simulink model "V.1.0.SystemsmModelling"  (R2020a)
settings: Solver=ode23t  StartTime=0.0  StopTime=2000  MaxStep=2000.0  RelTol=1e-3
values from neighbouring files (symbols this model uses):
  InitialTemp = 300    [Setup.m]
undefined symbols (not defined in the file or in its folder): commanded_mass_flow, compressor_time_constant, condenser_length, copper_density, environment_temperature, evaporator_length, ground_temperature, max_throat_area, max_throat_temperature, min_throat_area, min_throat_temperature, pipe_diameter, pipe_thickness, target_temperature, temperature_delta, u_sat
libraries: fl_lib x208, refrigeration_lib x90, fl_ps_legacy_lib x50, nesl_utility x45
(part 3 of 7)

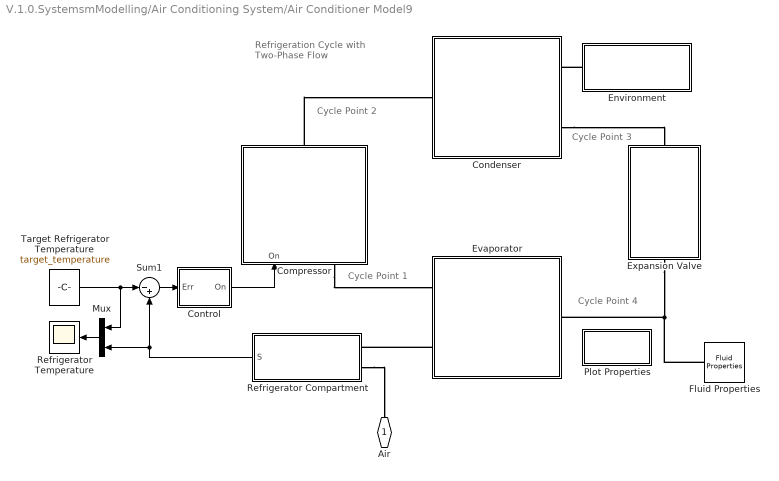
== system V.1.0.SystemsmModelling/Air Conditioning System/Air Conditioner Model9 ==
  note: Refrigeration Cycle
      | with Two-Phase Flow
  note: Cycle Point 1
  note: Cycle Point 3
  note: Cycle Point 2
  note: Cycle Point 4
  Compressor : Subsystem
      mask Display:
      | % Fading color
      | % Center to right
      | patch(sin(0.00*pi:0.05:1.10*pi),cos(0.00*pi:0.05:1.10*pi),[1;0.90;0.94]);
      | patch(sin(0.05*pi:0.05:0.95*pi),cos(0.05*pi:0.05:0.95*pi),[1;0.85;0.88]);
      | patch(sin(0.10*pi:0.05:0.90*pi),cos(0.10*pi:0.05:0.90*pi),[1;0.80;0.82]);
      | patch(sin(0.15*pi:0.05:0.85*pi),cos(0.15*pi:0.05:0.85*pi),[1;0.75;0.76]);
      | patch(sin(0.20*pi:0.05:0.80*pi),cos(0.20*pi:0.05:0.80*pi),[1;0.70;0.70]);
      | % Center to left
      | patch(sin(1.00*pi:0.05:2.00*pi),cos(1.00*pi:0.05:2.00*pi),[0.94;0.90;1]);
      | patch(sin(1.05*pi:0.05:1.95*pi),cos(1.05*pi:0.05:1.95*pi),[0.88;0.90;1]);
      | patch(sin(1.10*pi:0.05:1.90*pi),cos(1.10*pi:0.05:1.90*pi),[0.82;0.90;1]);
      | patch(sin(1.15*pi:0.05:1.85*pi),cos(1.15*pi:0.05:1.85*pi),[0.76;0.90;1]);
      | patch(sin(1.20*pi:0.05:1.80*pi),cos(1.20*pi:0.05:1.80*pi),[0.70;0.90;1]);
      | % Circle
      | plot(sin(0:0.1:2.2*pi),cos(0:0.1:2.2*pi));
      | % Angled lines
      | plot(sin([-0.6*pi/3 3.6*pi/8]),cos([-0.6*pi/3 3.6*pi/8]));
      | plot(sin([-0.6*pi/3 3.6*pi/8]),-cos([-0.6*pi/3 3.6*pi/8]));
      | plot(1.15*sin([-pi/4 3*pi/4]),1.15*cos([-pi/4 3*pi/4]));
      | % Arrow
      | patch([1.15*sin(-pi/4)+0.01;1.15*sin(3*pi/4)+0.01;1.15*sin(3*pi/4)-0.01;1.15*sin(-pi/4)-0.01],[1.15*cos(-pi/4)+0.01;1.15*cos(3*pi/4)+0.01;1.15*cos(3*pi/4)-0.01;1.15*cos(-pi/4)-0.01],[0;0;0])
      | patch([0.8*sin(3*pi/4)+0.05;1.15*sin(3*pi/4)+0.00;1.15*sin(3*pi/4)-0.00;0.8*sin(3*pi/4)-0.05],[0.8*cos(3*pi/4)+0.05;1.15*cos(3*pi/4)+0.00;1.15*cos(3*pi/4)-0.00;0.8*cos(3*pi/4)-0.05],[0;0;0])
      | % Points to set range for plotting area
      | color('white');plot(1.3,1.3);plot(-1.3,-1.3)
      | color('black');
      | 
      | port_label('LConn',1,'A');
      | port_label('RConn',1,'B');
      | port_label('input',1,'On');
  Condenser : Subsystem
      mask Display:
      | % Colored patches
      | % Center to right
      | patch(sin(0.0*pi:0.05:1.1*pi),cos(0.0*pi:0.05:1.1*pi),[1;0.58;0.58]);
      | patch(sin(0.1*pi:0.05:0.9*pi),cos(0.1*pi:0.05:0.9*pi),[1;0.64;0.64]);
      | patch(sin(0.2*pi:0.05:0.8*pi),cos(0.2*pi:0.05:0.8*pi),[1;0.70;0.70]);
      | % Center to left
      | patch(sin(1.0*pi:0.05:2.0*pi),cos(1.0*pi:0.05:2.0*pi),[1;0.52;0.52]);
      | patch(sin(1.1*pi:0.05:1.9*pi),cos(1.1*pi:0.05:1.9*pi),[1;0.46;0.46]);
      | patch(sin(1.2*pi:0.05:1.8*pi),cos(1.2*pi:0.05:1.8*pi),[1;0.40;0.40]);
      | % Circle
      | plot(sin(0:0.1:2.2*pi),cos(0:0.1:2.2*pi));
      | % 'M'
      | plot([0.5 0.5],[-1.2 0.5]);
      | plot([-0.5 -0.5],[-1.2 0.5]);
      | plot([0.5 0],[0.5 -0.2]);
      | plot([-0.5 0],[0.5 -0.2]);
      | % Plot points to set plot range
      | color('white');plot(1.3,1.3);plot(-1.3,-1.3)
      | color('black');
      | 
      | port_label('RConn',1,'A');
      | port_label('LConn',1,'T');
      | port_label('LConn',2,'B');
  Control : Subsystem
  Environment : Subsystem
      mask Display:
      | % Colored patch
      | patch([sin(0:0.1:1*pi)*0.25+0.4 sin(pi:0.1:2*pi)*0.25-0.4],[cos(0:0.1:1*pi) cos(pi:0.1:2*pi)],[1;0.9;0.9]);
      | % Outer rounded rectangle
      | plot(sin(0:0.1:1*pi)*0.25+0.4,cos(0:0.1:1*pi));
      | plot(sin(pi:0.1:2*pi)*0.25-0.4,cos(pi:0.1:2*pi));
      | plot([-0.4 0.4],[1 1]);
      | plot([-0.4 0.4],[-1 -1]);
      | % House frame
      | plot([-0.3 -0.3],[-0.866,0.866*0.2])
      | plot([0.3 0.3],[-0.866,0.866*0.2])
      | plot([0.3 0],[0.866*0.2, 0.866])
      | plot([-0.3 0],[0.866*0.2, 0.866])
      | plot([-0.3 0.3],[-0.866 -0.866])
      | plot([-0.3 0.3],[0.866 0.866]*0.2)
      | plot([-0.2 -0.04],[0.866 0.866]*0)
      | % Window
      | plot([-0.2 -0.04],[-1 -1]*0.2)
      | plot([-0.2 -0.04],[-1 -1]*0.4)
      | plot([-0.2 -0.2],[0 -0.4])
      | plot([-0.12 -0.12],[0 -0.4])
      | plot([-0.04 -0.04],[0 -0.4])
      | % Door
      | plot([0.05 0.05],[-0.866 -0.2])
      | plot([0.18 0.18],[-0.866 -0.2])
      | plot([0.05 0.18],[-0.2 -0.2])
      | patch([0.12 0.15 0.12 0.15],[-0.5 -0.5 -0.54 -0.54],[0;0;0])
      | % Outer boundary (so plot labels are visible)
      | color('white');plot(0.8660,0.8660);plot(-0.8660,-0.8660)
      | color('black');
      | port_label('LConn',1,'T');
  Evaporator : Subsystem
      mask Display:
      | % Fading color
      | % Center to right
      | patch(sin(0.00*pi:0.05:1.10*pi),cos(0.00*pi:0.05:1.10*pi),[0.58;0.70;1]);
      | patch(sin(0.05*pi:0.05:0.95*pi),cos(0.05*pi:0.05:0.95*pi),[0.63;0.75;1]);
      | patch(sin(0.10*pi:0.05:0.90*pi),cos(0.10*pi:0.05:0.90*pi),[0.66;0.80;1]);
      | patch(sin(0.15*pi:0.05:0.85*pi),cos(0.15*pi:0.05:0.85*pi),[0.69;0.85;1]);
      | patch(sin(0.20*pi:0.05:0.80*pi),cos(0.20*pi:0.05:0.80*pi),[0.70;0.90;1]);
      | % Center to left
      | patch(sin(1.00*pi:0.05:2.00*pi),cos(1.00*pi:0.05:2.00*pi),[0.52;0.60;1]);
      | patch(sin(1.05*pi:0.05:1.95*pi),cos(1.05*pi:0.05:1.95*pi),[0.49;0.55;1]);
      | patch(sin(1.10*pi:0.05:1.90*pi),cos(1.10*pi:0.05:1.90*pi),[0.46;0.50;1]);
      | patch(sin(1.15*pi:0.05:1.85*pi),cos(1.15*pi:0.05:1.85*pi),[0.43;0.45;1]);
      | patch(sin(1.20*pi:0.05:1.80*pi),cos(1.20*pi:0.05:1.80*pi),[0.40;0.40;1]);
      | % Circle
      | plot(sin(0:0.1:2.2*pi),cos(0:0.1:2.2*pi));
      | % 'M'
      | plot([0.5 0.5],[-1.2 0.5]);
      | plot([-0.5 -0.5],[-1.2 0.5]);
      | plot([0.5 0],[0.5 -0.2]);
      | plot([-0.5 0],[0.5 -0.2]);
      | % Plot points to set plotting range
      | color('white');plot(1.3,1.3);plot(-1.3,-1.3)
      | color('black');
      | 
      | port_label('LConn',1,'A');
      | port_label('RConn',1,'B');
      | port_label('RConn',2,'T');
  Expansion Valve : Subsystem
      mask Display:
      | % Colored patches
      | patch([-1 -1 0],[0.5 -0.5 0],[1;0.4;0.4]);
      | patch([1 1 0],[0.5 -0.5 0],[0.4;0.4;1]);
      | % Valve
      | plot([1 1],[0.5 -0.5]);
      | plot([-1 -1],[0.5 -0.5]);
      | plot([-1 1],[0.5 -0.5]);
      | plot([-1 1],[-0.5 0.5]);
      | % Arrow
      | patch([1.15*sin(-pi/4-0.01);1.15*sin(-pi/4+0.01);1*sin(3*pi/4-0.01);1*sin(3*pi/4+0.01)],[1.15*cos(-pi/4-0.01);1.15*cos(-pi/4+0.01);1*cos(3*pi/4-0.01);1*cos(3*pi/4+0.01)],[0;0;0])
      | patch([0.8*sin(3*pi/4+0.07);1.15*sin(3*pi/4+0.00);1.15*sin(3*pi/4-0.00);0.8*sin(3*pi/4-0.07)],[0.8*cos(3*pi/4+0.07);1.15*cos(3*pi/4+0.00);1.15*cos(3*pi/4-0.00);0.8*cos(3*pi/4-0.07)],[0;0;0])
      | % Plot outer points to set plot range
      | color('white'); plot(-1.3,0); plot(1.3,0);
      | color('black');
      | port_label('LConn',1,'A');
      | port_label('RConn',1,'B');
  Fluid Properties : refrigeration_lib/Fluid Properties  p_TLU=p_TLU MPa  u_TLU=u_TLU kJ/kg  v_TLU=v_TLU m^3/kg  T_TLU=T_TLU K  mu_TLU=mu_TLU s*uPa  k_TLU=k_TLU W/(m*K)  Pr_TLU=Pr_TLU  u_liq=u_sat(:,1) kJ/kg  u_vap=u_sat(:,2) kJ/kg
      settings: InternalSimscapePortConfiguration="{\"Bottom\":[],\"Left\":[],\"Right\":[{\"id\":\"A\",\"label\":\"\",\"type\":\"refrigeration.refrigeration\"}],\"Top\":[]}"
  Mux : Mux  Inputs=2
  Plot Properties : Subsystem
      settings: OpenFcn=plotFluidProperties()
      mask Display: disp('Plot Fluid\nProperties');
  Refrigerator Compartment : Subsystem
      mask Display:
      | % Color
      | patch([sin(0:0.1:1*pi)*0.25+0.4 sin(pi:0.1:2*pi)*0.25-0.4],[cos(0:0.1:1*pi) cos(pi:0.1:2*pi)],[0.70;0.90;1]);
      | % Outer rounded rectangle
      | plot(sin(pi:0.1:2*pi)*0.25-0.4,cos(pi:0.1:2*pi));
      | plot(sin(0:0.1:1*pi)*0.25+0.4,cos(0:0.1:1*pi));
      | plot(sin(pi:0.1:2*pi)*0.25-0.4,cos(pi:0.1:2*pi));
      | plot([-0.4 0.4],[1 1]);
      | plot([-0.4 0.4],[-1 -1]);
      | % Outer points to set size of plot range
      | color('white');plot(0.8660,0.8660);plot(-0.8660,-0.8660)
      | color('black');
      | % Snowflake
      | plot([0 0],[0.8 -0.8]);
      | plot([0 0.1],[0.5 0.7]);
      | plot([0 -0.1],[0.5 0.7]);
      | plot([0 0.1],[-0.5 -0.7]);
      | plot([0 -0.1],[-0.5 -0.7]);
      | plot(0.3*sin([pi/3 4*pi/3]),1*cos([pi/3 4*pi/3]));
      | plot([0.22*sin(pi/3) 0.25*sin(pi/4)],[0.7*cos(pi/3) 0.84*cos(pi/4)]);
      | plot([0.22*sin(pi/3) 0.25*sin(pi/2)],[0.7*cos(pi/3) 0.325*cos(pi/4)]);
      | plot([0.22*sin(pi/3) 0.25*sin(pi/4)],[-0.7*cos(pi/3) -0.84*cos(pi/4)]);
      | plot([0.22*sin(pi/3) 0.25*sin(pi/2)],[-0.7*cos(pi/3) -0.325*cos(pi/4)]);
      | plot(-0.3*sin([pi/3 4*pi/3]),1*cos([pi/3 4*pi/3]));
      | plot([-0.22*sin(pi/3) -0.25*sin(pi/4)],[0.7*cos(pi/3) 0.84*cos(pi/4)]);
      | plot([-0.22*sin(pi/3) -0.25*sin(pi/2)],[0.7*cos(pi/3) 0.325*cos(pi/4)]);
      | plot([-0.22*sin(pi/3) -0.25*sin(pi/4)],[-0.7*cos(pi/3) -0.84*cos(pi/4)]);
      | plot([-0.22*sin(pi/3) -0.25*sin(pi/2)],[-0.7*cos(pi/3) -0.325*cos(pi/4)]);
      | plot([0 0.1],[-0.5 -0.7]);
      | plot([0 -0.1],[-0.5 -0.7]);
      | % Labels
      | port_label('LConn',1,'T');
      | port_label('output',1,'S');
  Refrigerator Temperature : Scope
  Sum1 : Sum  Inputs=|-+
  Target Refrigerator Temperature : Constant  Value=target_temperature
  Air : PMIOPort  Side=Left
  wires:
  Control/1(On) -> Compressor/1(On)
  Refrigerator Compartment/1(S) -> Mux/2, Sum1/2
  Target Refrigerator Temperature/1 -> Sum1/1, Mux/1
  Mux/1 -> Refrigerator Temperature/1
  Sum1/1 -> Control/1(Err)
  connections:
  Expansion Valve/RConn1 -- Fluid Properties/RConn1 -- Evaporator/LConn1
  Environment/LConn1 -- Condenser/LConn1
  Evaporator/RConn2 -- Refrigerator Compartment/LConn1
  Compressor/LConn1 -- Evaporator/RConn1
  Condenser/LConn2 -- Expansion Valve/LConn1
  Compressor/RConn1 -- Condenser/RConn1
  Refrigerator Compartment/LConn2 -- Air/RConn1

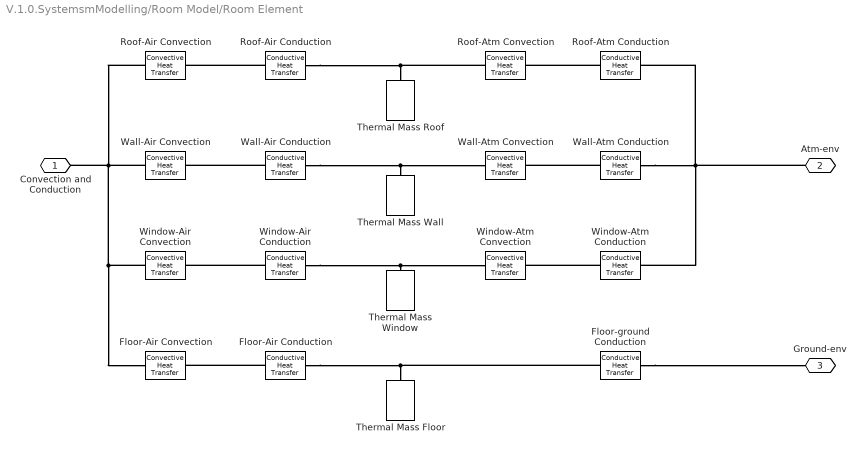
== system V.1.0.SystemsmModelling/Room Model/Room Element  ==
  " Wall-Air Conduction" : fl_lib/Thermal/Thermal Elements/Conductive Heat Transfer  area=375 m^2  thickness=0.2 m  th_cond=0.15 W/(m*K)  T_specify=off  T_priority=None  T=0 K  T_nominal_specify=off  T_nominal_unit=K  T_nominal_value=1  Q_specify=off  Q_priority=None  Q=0 W  Q_nominal_specify=off  Q_nominal_unit=W  Q_nominal_value=1
  " Wall-Atm Conduction" : fl_lib/Thermal/Thermal Elements/Conductive Heat Transfer  area=375 m^2  thickness=0.2 m  th_cond=0.15 W/(m*K)  T_specify=off  T_priority=None  T=0 K  T_nominal_specify=off  T_nominal_unit=K  T_nominal_value=1  Q_specify=off  Q_priority=None  Q=0 W  Q_nominal_specify=off  Q_nominal_unit=W  Q_nominal_value=1
  " Window-Air Conduction" : fl_lib/Thermal/Thermal Elements/Conductive Heat Transfer  area=25 m^2  thickness=0.2 m  th_cond=0.96 W/(m*K)  T_specify=off  T_priority=None  T=0 K  T_nominal_specify=off  T_nominal_unit=K  T_nominal_value=1  Q_specify=off  Q_priority=None  Q=0 W  Q_nominal_specify=off  Q_nominal_unit=W  Q_nominal_value=1
  " Window-Atm Conduction" : fl_lib/Thermal/Thermal Elements/Conductive Heat Transfer  area=25 m^2  thickness=0.2 m  th_cond=0.96 W/(m*K)  T_specify=off  T_priority=None  T=0 K  T_nominal_specify=off  T_nominal_unit=K  T_nominal_value=1  Q_specify=off  Q_priority=None  Q=0 W  Q_nominal_specify=off  Q_nominal_unit=W  Q_nominal_value=1
  Floor-Air Conduction : fl_lib/Thermal/Thermal Elements/Conductive Heat Transfer  area=25 m^2  thickness=0.2 m  th_cond=0.96 W/(m*K)  T_specify=off  T_priority=None  T=0 K  T_nominal_specify=off  T_nominal_unit=K  T_nominal_value=1  Q_specify=off  Q_priority=None  Q=0 W  Q_nominal_specify=off  Q_nominal_unit=W  Q_nominal_value=1
  Floor-Air Convection : fl_lib/Thermal/Thermal Elements/Convective Heat Transfer  area=20 m^2  heat_tr_coeff=3.3 W/(m^2 * K)  T_specify=off  T_priority=None  T=0 K  T_nominal_specify=off  T_nominal_unit=K  T_nominal_value=1  Q_specify=off  Q_priority=None  Q=0 W  Q_nominal_specify=off  Q_nominal_unit=W  Q_nominal_value=1
  Floor-ground Conduction : fl_lib/Thermal/Thermal Elements/Conductive Heat Transfer  area=25 m^2  thickness=0.2 m  th_cond=0.96 W/(m*K)  T_specify=off  T_priority=None  T=0 K  T_nominal_specify=off  T_nominal_unit=K  T_nominal_value=1  Q_specify=off  Q_priority=None  Q=0 W  Q_nominal_specify=off  Q_nominal_unit=W  Q_nominal_value=1
  Roof-Air Conduction : fl_lib/Thermal/Thermal Elements/Conductive Heat Transfer  area=100 m^2  thickness=0.2 m  th_cond=0.12 W/(m*K)  T_specify=off  T_priority=None  T=0 K  T_nominal_specify=off  T_nominal_unit=K  T_nominal_value=1  Q_specify=off  Q_priority=None  Q=0 W  Q_nominal_specify=off  Q_nominal_unit=W  Q_nominal_value=1
  Roof-Air Convection : fl_lib/Thermal/Thermal Elements/Convective Heat Transfer  area=100 m^2  heat_tr_coeff=20 W/(m^2 * K)  T_specify=off  T_priority=None  T=0 K  T_nominal_specify=off  T_nominal_unit=K  T_nominal_value=1  Q_specify=off  Q_priority=None  Q=0 W  Q_nominal_specify=off  Q_nominal_unit=W  Q_nominal_value=1
  Roof-Atm Conduction : fl_lib/Thermal/Thermal Elements/Conductive Heat Transfer  area=100 m^2  thickness=0.2 m  th_cond=0.12 W/(m*K)  T_specify=off  T_priority=None  T=0 K  T_nominal_specify=off  T_nominal_unit=K  T_nominal_value=1  Q_specify=off  Q_priority=None  Q=0 W  Q_nominal_specify=off  Q_nominal_unit=W  Q_nominal_value=1
  Roof-Atm Convection : fl_lib/Thermal/Thermal Elements/Convective Heat Transfer  area=100 m^2  heat_tr_coeff=20 W/(m^2 * K)  T_specify=off  T_priority=None  T=0 K  T_nominal_specify=off  T_nominal_unit=K  T_nominal_value=1  Q_specify=off  Q_priority=None  Q=0 W  Q_nominal_specify=off  Q_nominal_unit=W  Q_nominal_value=1
  Thermal Mass Floor : fl_lib/Thermal/Thermal Elements/Thermal Mass  mass=48 kg  sp_heat=840.7 J/kg/K  T_specify=on  T_priority=High  T=InitialTemp K  T_nominal_specify=off  T_nominal_unit=K  T_nominal_value=1  Q_specify=off  Q_priority=None  Q=0 W  Q_nominal_specify=off  Q_nominal_unit=W  Q_nominal_value=1
  Thermal Mass Roof : fl_lib/Thermal/Thermal Elements/Thermal Mass  mass=48 kg  sp_heat=853.7 J/kg/K  T_specify=on  T_priority=High  T=InitialTemp K  T_nominal_specify=off  T_nominal_unit=K  T_nominal_value=1  Q_specify=off  Q_priority=None  Q=0 W  Q_nominal_specify=off  Q_nominal_unit=W  Q_nominal_value=1
  Thermal Mass Wall : fl_lib/Thermal/Thermal Elements/Thermal Mass  mass=180 kg  sp_heat=868.2 J/kg/K  T_specify=on  T_priority=High  T=InitialTemp K  T_nominal_specify=off  T_nominal_unit=K  T_nominal_value=1  Q_specify=off  Q_priority=None  Q=0 W  Q_nominal_specify=off  Q_nominal_unit=W  Q_nominal_value=1
  Thermal Mass Window : fl_lib/Thermal/Thermal Elements/Thermal Mass  mass=11 kg  sp_heat=840 J/kg/K  T_specify=on  T_priority=High  T=InitialTemp K  T_nominal_specify=off  T_nominal_unit=K  T_nominal_value=1  Q_specify=off  Q_priority=None  Q=0 W  Q_nominal_specify=off  Q_nominal_unit=W  Q_nominal_value=1
  Wall-Air Convection : fl_lib/Thermal/Thermal Elements/Convective Heat Transfer  area=375 m^2  heat_tr_coeff=20 W/(m^2 * K)  T_specify=off  T_priority=None  T=0 K  T_nominal_specify=off  T_nominal_unit=K  T_nominal_value=1  Q_specify=off  Q_priority=None  Q=0 W  Q_nominal_specify=off  Q_nominal_unit=W  Q_nominal_value=1
  Wall-Atm Convection : fl_lib/Thermal/Thermal Elements/Convective Heat Transfer  area=375 m^2  heat_tr_coeff=20 W/(m^2 * K)  T_specify=off  T_priority=None  T=0 K  T_nominal_specify=off  T_nominal_unit=K  T_nominal_value=1  Q_specify=off  Q_priority=None  Q=0 W  Q_nominal_specify=off  Q_nominal_unit=W  Q_nominal_value=1
  Window-Air Convection : fl_lib/Thermal/Thermal Elements/Convective Heat Transfer  area=25 m^2  heat_tr_coeff=3.3 W/(m^2 * K)  T_specify=off  T_priority=None  T=0 K  T_nominal_specify=off  T_nominal_unit=K  T_nominal_value=1  Q_specify=off  Q_priority=None  Q=0 W  Q_nominal_specify=off  Q_nominal_unit=W  Q_nominal_value=1
  Window-Atm Convection : fl_lib/Thermal/Thermal Elements/Convective Heat Transfer  area=25 m^2  heat_tr_coeff=3.3 W/(m^2 * K)  T_specify=off  T_priority=None  T=0 K  T_nominal_specify=off  T_nominal_unit=K  T_nominal_value=1  Q_specify=off  Q_priority=None  Q=0 W  Q_nominal_specify=off  Q_nominal_unit=W  Q_nominal_value=1
  Convection and Conduction : PMIOPort  Side=Left
  Atm-env : PMIOPort  Port=2  Side=Left
  Ground-env : PMIOPort  Port=3  Side=Left
  connections:
  " Window-Atm Conduction"/RConn1 -- Window-Atm Convection/LConn1
  Floor-ground Conduction/LConn1 -- Ground-env/RConn1
  Roof-Air Conduction/RConn1 -- Roof-Air Convection/LConn1
  Floor-Air Conduction/LConn1 -- Floor-ground Conduction/RConn1 -- Thermal Mass Floor/LConn1
  " Wall-Atm Conduction"/LConn1 -- Atm-env/RConn1 -- Roof-Atm Conduction/LConn1 -- " Window-Atm Conduction"/LConn1
  Roof-Air Convection/RConn1 -- Convection and Conduction/RConn1 -- Window-Air Convection/RConn1 -- Floor-Air Convection/RConn1 -- Wall-Air Convection/RConn1
  Roof-Atm Convection/RConn1 -- Roof-Air Conduction/LConn1 -- Thermal Mass Roof/LConn1
  Roof-Atm Conduction/RConn1 -- Roof-Atm Convection/LConn1
  " Wall-Air Conduction"/LConn1 -- Wall-Atm Convection/RConn1 -- Thermal Mass Wall/LConn1
  " Window-Air Conduction"/LConn1 -- Window-Atm Convection/RConn1 -- Thermal Mass Window/LConn1
  " Wall-Atm Conduction"/RConn1 -- Wall-Atm Convection/LConn1
  " Wall-Air Conduction"/RConn1 -- Wall-Air Convection/LConn1
  " Window-Air Conduction"/RConn1 -- Window-Air Convection/LConn1
  Floor-Air Conduction/RConn1 -- Floor-Air Convection/LConn1

== system V.1.0.SystemsmModelling/Air Conditioning System/Air Conditioner Model/Compressor ==
  On : Inport
  Commanded Mass Flow Rate : Gain  Gain=commanded_mass_flow
  Compressor Lag : TransferFcn  Numerator=[(9/compressor_time_constant)^2]  Denominator=[1, 2*(9/compressor_time_constant), (9/compressor_time_constant)^2]
  Controlled Mass Flow Rate Source : refrigeration_lib/Controlled Mass Flow Rate Source  S=pi*pipe_diameter^2/4 m^2  L=0.1 m  mdot_specify=off  mdot_priority=High  mdot=0 kg/s  mdot_nominal_specify=off  mdot_nominal_unit=kg/s  mdot_nominal_value=1  phi_A_specify=off  phi_A_priority=High  phi_A=0 kW  phi_A_nominal_specify=off  phi_A_nominal_unit=kW  phi_A_nominal_value=1  phi_B_specify=off  phi_B_priority=High  phi_B=0 kW  phi_B_nominal_specify=off  phi_B_nominal_unit=kW  phi_B_nominal_value=1  u_AI_specify=off  u_AI_priority=High  u_AI=396.921741345 kJ/kg  u_AI_nominal_specify=off  u_AI_nominal_unit=kJ/kg  u_AI_nominal_value=1  v_A_specify=off  v_A_priority=High  v_A=0.230606289431 m^3/kg  v_A_nominal_specify=off  v_A_nominal_unit=m^3/kg  v_A_nominal_value=1  u_BI_specify=off  u_BI_priority=High  u_BI=396.921741345 kJ/kg  u_BI_nominal_specify=off  u_BI_nominal_unit=kJ/kg  u_BI_nominal_value=1  v_B_specify=off  v_B_priority=High  v_B=0.230606289431 m^3/kg  v_B_nominal_specify=off  v_B_nominal_unit=m^3/kg  v_B_nominal_value=1  u_2_specify=off  u_2_priority=High  u_2=396.921741345 kJ/kg  u_2_nominal_specify=off  u_2_nominal_unit=kJ/kg  u_2_nominal_value=1  u_3_specify=off  u_3_priority=High  u_3=396.921741345 kJ/kg  u_3_nominal_specify=off  u_3_nominal_unit=kJ/kg  u_3_nominal_value=1
      settings: InternalSimscapePortConfiguration="{\"Bottom\":[],\"Left\":[{\"id\":\"A\",\"label\":\"A\",\"type\":\"refrigeration.refrigeration\"},{\"id\":\"M\",\"label\":\"M\",\"type\":\"input\"}],\"Right\":[{\"id\":\"B\",\"label\":\"B\",\"type\":\"refrigeration.refrigeration\"},{\"id\":\"W\",\"label\":\"W\",\"type\":\"output\"}],\"Top\":[]}"
  Simulink-PS Converter : nesl_utility/Simulink-PS Converter  PhysicalDomain=network_engine_domain  SubClassName=ps_input  LeftPortType=input  RightPortType=output  PseudoPeriodic=off  Frequencies=[]  NoiseDistribution=none  NoiseParameters=[]  Unit=kg/s  AffineConversion=off  FilteringAndDerivatives=zero  SimscapeFilterOrder=1  InputFilterTimeConstant=0.001  UdotUserProvided=1
  B : PMIOPort  Side=Right
  A : PMIOPort  Port=2  Side=Left
  wires:
  Compressor Lag/1 -> Simulink-PS Converter/1
  Commanded Mass Flow Rate/1 -> Compressor Lag/1
  On/1 -> Commanded Mass Flow Rate/1
  connections:
  Controlled Mass Flow Rate Source/RConn1 -- B/RConn1
  Controlled Mass Flow Rate Source/LConn2 -- Simulink-PS Converter/RConn1
  A/RConn1 -- Controlled Mass Flow Rate Source/LConn1

== system V.1.0.SystemsmModelling/Air Conditioning System/Air Conditioner Model/Condenser ==
  Condenser Conduction : fl_lib/Thermal/Thermal Elements/Conductive Heat Transfer  area=pi*pipe_diameter*condenser_length m^2  thickness=pipe_thickness m  th_cond=copper_conductivity W/(m*K)  T_specify=off  T_priority=High  T=0 K  T_nominal_specify=off  T_nominal_unit=K  T_nominal_value=1  Q_specify=off  Q_priority=High  Q=0 J/s  Q_nominal_specify=off  Q_nominal_unit=W  Q_nominal_value=1
  Condenser Copper : fl_lib/Thermal/Thermal Elements/Thermal Mass  mass=pi*pipe_diameter*condenser_length*pipe_thickness*copper_density kg  sp_heat=copper_specific_heat J/kg/K  T_specify=on  T_priority=High  T=environment_temperature K  T_nominal_specify=off  T_nominal_unit=K  T_nominal_value=1  Q_specify=off  Q_priority=High  Q=0 J/s  Q_nominal_specify=off  Q_nominal_unit=W  Q_nominal_value=1
  Condenser Pipe : refrigeration_lib/Pipe  L=condenser_length m  S=pi*pipe_diameter^2/4 m^2  Dh=pipe_diameter m  fs=64  La=0.1*condenser_length m  eps=15e-6 m  Re_lam=2000  Re_tur=4000  J_smooth=5 kg/m^2/s  p_0=charge_pressure MPa  T_0=-1 K  x_0=initial_quality  mdot_A_specify=off  mdot_A_priority=High  mdot_A=0 kg/s  mdot_A_nominal_specify=off  mdot_A_nominal_unit=kg/s  mdot_A_nominal_value=1  mdot_B_specify=off  mdot_B_priority=High  mdot_B=0 kg/s  mdot_B_nominal_specify=off  mdot_B_nominal_unit=kg/s  mdot_B_nominal_value=1  phi_A_specify=off  phi_A_priority=High  phi_A=0 kW  phi_A_nominal_specify=off  phi_A_nominal_unit=kW  phi_A_nominal_value=1  phi_B_specify=off  phi_B_priority=High  phi_B=0 kW  phi_B_nominal_specify=off  phi_B_nominal_unit=kW  phi_B_nominal_value=1  v_A_specify=off  v_A_priority=High  v_A=0.230606289431 m^3/kg  v_A_nominal_specify=off  v_A_nominal_unit=m^3/kg  v_A_nominal_value=1  v_B_specify=off  v_B_priority=High  v_B=0.230606289431 m^3/kg  v_B_nominal_specify=off  v_B_nominal_unit=m^3/kg  v_B_nominal_value=1  p_I_specify=off  p_I_priority=High  p_I=0.101325 MPa  p_I_nominal_specify=off  p_I_nominal_unit=MPa  p_I_nominal_value=1  u_I_specify=off  u_I_priority=High  u_I=396.921741345 kJ/kg  u_I_nominal_specify=off  u_I_nominal_unit=kJ/kg  u_I_nominal_value=1  v_I_specify=off  v_I_priority=High  v_I=0.230606289431 m^3/kg  v_I_nominal_specify=off  v_I_nominal_unit=m^3/kg  v_I_nominal_value=1  q_T_specify=off  q_T_priority=High  q_T=0 kW  q_T_nominal_specify=off  q_T_nominal_unit=kW  q_T_nominal_value=1  Ff_A_specify=off  Ff_A_priority=High  Ff_A=0 N  Ff_A_nominal_specify=off  Ff_A_nominal_unit=N  Ff_A_nominal_value=1  Ff_B_specify=off  Ff_B_priority=High  Ff_B=0 N  Ff_B_nominal_specify=off  Ff_B_nominal_unit=N  Ff_B_nominal_value=1  ev_I_specify=off  ev_I_priority=High  ev_I=1.7212095226213e+3 kJ/m^3  ev_I_nominal_specify=off  ev_I_nominal_unit=kJ/m^3  ev_I_nominal_value=1  mdot_I_specify=off  mdot_I_priority=High  mdot_I=0 kg/s  mdot_I_nominal_specify=off  mdot_I_nominal_unit=kg/s  mdot_I_nominal_value=1  Nu_I_specify=off  Nu_I_priority=High  Nu_I=0  Nu_I_nominal_specify=off  Nu_I_nominal_unit=1  Nu_I_nominal_value=1
      settings: InternalSimscapePortConfiguration="{\"Bottom\":[],\"Left\":[{\"id\":\"A\",\"label\":\"A\",\"type\":\"refrigeration.refrigeration\"},{\"id\":\"T\",\"label\":\"T\",\"type\":\"foundation.thermal.thermal\"}],\"Right\":[{\"id\":\"B\",\"label\":\"B\",\"type\":\"refrigeration.refrigeration\"}],\"Top\":[]}"
  T : PMIOPort  Side=Left
  B : PMIOPort  Port=2  Side=Left
  A : PMIOPort  Port=3  Side=Right
  connections:
  Condenser Conduction/LConn1 -- Condenser Pipe/LConn2 -- Condenser Copper/LConn1
  T/RConn1 -- Condenser Conduction/RConn1
  B/RConn1 -- Condenser Pipe/RConn1
  Condenser Pipe/LConn1 -- A/RConn1

== system V.1.0.SystemsmModelling/Air Conditioning System/Air Conditioner Model/Control ==
  Err : Inport
  Relay : Relay  OnSwitchValue=temperature_delta  OffSwitchValue=-temperature_delta
  On : Outport
  wires:
  Err/1 -> Relay/1
  Relay/1 -> On/1

== system V.1.0.SystemsmModelling/Air Conditioning System/Air Conditioner Model/Environment ==
  Condenser Convection : fl_lib/Thermal/Thermal Elements/Convective Heat Transfer  area=fin_area m^2  heat_tr_coeff=fin_convection_coefficient W/(m^2 * K)  T_specify=off  T_priority=High  T=0 K  T_nominal_specify=off  T_nominal_unit=K  T_nominal_value=1  Q_specify=off  Q_priority=High  Q=0 J/s  Q_nominal_specify=off  Q_nominal_unit=W  Q_nominal_value=1
  Constant : Constant  Value=environment_temperature
  Ideal Temperature Source : fl_lib/Thermal/Thermal Sources/Controlled Temperature Source
  Simulink-PS Converter : nesl_utility/Simulink-PS Converter  PhysicalDomain=network_engine_domain  SubClassName=ps_input  LeftPortType=input  RightPortType=output  PseudoPeriodic=off  Frequencies=[]  NoiseDistribution=none  NoiseParameters=[]  Unit=K  AffineConversion=off  FilteringAndDerivatives=zero  SimscapeFilterOrder=1  InputFilterTimeConstant=0.001  UdotUserProvided=1
  Thermal Reference : fl_lib/Thermal/Thermal Elements/Thermal Reference
  T : PMIOPort  Side=Left
  wires:
  Constant/1 -> Simulink-PS Converter/1
  connections:
  Condenser Convection/RConn1 -- Ideal Temperature Source/LConn1
  Condenser Convection/LConn1 -- T/RConn1
  Ideal Temperature Source/RConn1 -- Simulink-PS Converter/RConn1
  Ideal Temperature Source/RConn2 -- Thermal Reference/LConn1

== system V.1.0.SystemsmModelling/Air Conditioning System/Air Conditioner Model/Evaporator ==
  Evaporator Conduction : fl_lib/Thermal/Thermal Elements/Conductive Heat Transfer  area=pi*pipe_diameter*evaporator_length m^2  thickness=pipe_thickness m  th_cond=copper_conductivity W/(m*K)  T_specify=off  T_priority=High  T=0 K  T_nominal_specify=off  T_nominal_unit=K  T_nominal_value=1  Q_specify=off  Q_priority=High  Q=0 J/s  Q_nominal_specify=off  Q_nominal_unit=W  Q_nominal_value=1
  Evaporator Copper : fl_lib/Thermal/Thermal Elements/Thermal Mass  mass=pi*pipe_diameter*evaporator_length*pipe_thickness*copper_density kg  sp_heat=copper_specific_heat J/kg/K  T_specify=on  T_priority=High  T=target_temperature K  T_nominal_specify=off  T_nominal_unit=K  T_nominal_value=1  Q_specify=off  Q_priority=High  Q=0 J/s  Q_nominal_specify=off  Q_nominal_unit=W  Q_nominal_value=1
  Evaporator Pipe : refrigeration_lib/Pipe  L=evaporator_length m  S=pi*pipe_diameter^2/4 m^2  Dh=pipe_diameter m  fs=64  La=0.1*evaporator_length m  eps=15e-6 m  Re_lam=2000  Re_tur=4000  J_smooth=5 kg/m^2/s  p_0=charge_pressure MPa  T_0=-1 K  x_0=initial_quality  mdot_A_specify=off  mdot_A_priority=High  mdot_A=0 kg/s  mdot_A_nominal_specify=off  mdot_A_nominal_unit=kg/s  mdot_A_nominal_value=1  mdot_B_specify=off  mdot_B_priority=High  mdot_B=0 kg/s  mdot_B_nominal_specify=off  mdot_B_nominal_unit=kg/s  mdot_B_nominal_value=1  phi_A_specify=off  phi_A_priority=High  phi_A=0 kW  phi_A_nominal_specify=off  phi_A_nominal_unit=kW  phi_A_nominal_value=1  phi_B_specify=off  phi_B_priority=High  phi_B=0 kW  phi_B_nominal_specify=off  phi_B_nominal_unit=kW  phi_B_nominal_value=1  v_A_specify=off  v_A_priority=High  v_A=0.230606289431 m^3/kg  v_A_nominal_specify=off  v_A_nominal_unit=m^3/kg  v_A_nominal_value=1  v_B_specify=off  v_B_priority=High  v_B=0.230606289431 m^3/kg  v_B_nominal_specify=off  v_B_nominal_unit=m^3/kg  v_B_nominal_value=1  p_I_specify=off  p_I_priority=High  p_I=0.101325 MPa  p_I_nominal_specify=off  p_I_nominal_unit=MPa  p_I_nominal_value=1  u_I_specify=off  u_I_priority=High  u_I=396.921741345 kJ/kg  u_I_nominal_specify=off  u_I_nominal_unit=kJ/kg  u_I_nominal_value=1  v_I_specify=off  v_I_priority=High  v_I=0.230606289431 m^3/kg  v_I_nominal_specify=off  v_I_nominal_unit=m^3/kg  v_I_nominal_value=1  q_T_specify=off  q_T_priority=High  q_T=0 kW  q_T_nominal_specify=off  q_T_nominal_unit=kW  q_T_nominal_value=1  Ff_A_specify=off  Ff_A_priority=High  Ff_A=0 N  Ff_A_nominal_specify=off  Ff_A_nominal_unit=N  Ff_A_nominal_value=1  Ff_B_specify=off  Ff_B_priority=High  Ff_B=0 N  Ff_B_nominal_specify=off  Ff_B_nominal_unit=N  Ff_B_nominal_value=1  ev_I_specify=off  ev_I_priority=High  ev_I=1.7212095226213e+3 kJ/m^3  ev_I_nominal_specify=off  ev_I_nominal_unit=kJ/m^3  ev_I_nominal_value=1  mdot_I_specify=off  mdot_I_priority=High  mdot_I=0 kg/s  mdot_I_nominal_specify=off  mdot_I_nominal_unit=kg/s  mdot_I_nominal_value=1  Nu_I_specify=off  Nu_I_priority=High  Nu_I=0  Nu_I_nominal_specify=off  Nu_I_nominal_unit=1  Nu_I_nominal_value=1
      settings: InternalSimscapePortConfiguration="{\"Bottom\":[],\"Left\":[{\"id\":\"A\",\"label\":\"A\",\"type\":\"refrigeration.refrigeration\"},{\"id\":\"T\",\"label\":\"T\",\"type\":\"foundation.thermal.thermal\"}],\"Right\":[{\"id\":\"B\",\"label\":\"B\",\"type\":\"refrigeration.refrigeration\"}],\"Top\":[]}"
  A : PMIOPort  Side=Left
  B : PMIOPort  Port=2  Side=Right
  T : PMIOPort  Port=3  Side=Right
  connections:
  Evaporator Conduction/RConn1 -- T/RConn1
  Evaporator Copper/LConn1 -- Evaporator Pipe/LConn2 -- Evaporator Conduction/LConn1
  Evaporator Pipe/RConn1 -- B/RConn1
  Evaporator Pipe/LConn1 -- A/RConn1

== system V.1.0.SystemsmModelling/Air Conditioning System/Air Conditioner Model/Expansion Valve ==
  Controlled Local Restriction : refrigeration_lib/Controlled Local Restriction  Cd=0.7  L=0.1 m  S=pi*pipe_diameter^2/4 m^2
      settings: InternalSimscapePortConfiguration="{\"Bottom\":[],\"Left\":[{\"id\":\"A\",\"label\":\"A\",\"type\":\"refrigeration.refrigeration\"},{\"id\":\"Sr\",\"label\":\"S\",\"type\":\"input\"}],\"Right\":[{\"id\":\"B\",\"label\":\"B\",\"type\":\"refrigeration.refrigeration\"}],\"Top\":[]}"
  Cycle Sensor 4 : Subsystem
  Display : Display
  Mass Flow Sensor : Subsystem
  PS-Simulink Converter : nesl_utility/PS-Simulink Converter  PhysicalDomain=network_engine_domain  SubClassName=ps_output  LeftPortType=input  RightPortType=output  PseudoPeriodic=off  Frequencies=[]  Unit=inherit  AffineConversion=off
  Valve Control : Subsystem
  A : PMIOPort  Side=Left
  B : PMIOPort  Port=2  Side=Right
  wires:
  PS-Simulink Converter/1 -> Display/1
  connections:
  B/RConn1 -- Cycle Sensor 4/LConn1 -- Mass Flow Sensor/RConn1
  Controlled Local Restriction/LConn1 -- A/RConn1
  Controlled Local Restriction/RConn1 -- Mass Flow Sensor/LConn1
  Controlled Local Restriction/LConn2 -- PS-Simulink Converter/LConn1 -- Valve Control/LConn1
  Cycle Sensor 4/RConn1 -- Valve Control/RConn1

== system V.1.0.SystemsmModelling/Air Conditioning System/Air Conditioner Model/Plot Properties ==

== system V.1.0.SystemsmModelling/Air Conditioning System/Air Conditioner Model/Refrigerator Compartment ==
  Environment Temperature : Subsystem
  Evaporator Convection : fl_lib/Thermal/Thermal Elements/Convective Heat Transfer  area=interior_surface_area m^2  heat_tr_coeff=natural_convection_coefficient W/(m^2 * K)  T_specify=off  T_priority=High  T=0 K  T_nominal_specify=off  T_nominal_unit=K  T_nominal_value=1  Q_specify=off  Q_priority=High  Q=0 J/s  Q_nominal_specify=off  Q_nominal_unit=W  Q_nominal_value=1
  Heat Flow Sensor : Subsystem
  Polyurethane Foam Conduction : fl_lib/Thermal/Thermal Elements/Conductive Heat Transfer  area=interior_surface_area m^2  thickness=foam_thickness m  th_cond=foam_conductivity W/(m*K)  T_specify=off  T_priority=High  T=0 K  T_nominal_specify=off  T_nominal_unit=K  T_nominal_value=1  Q_specify=off  Q_priority=High  Q=0 J/s  Q_nominal_specify=off  Q_nominal_unit=W  Q_nominal_value=1
  Refrigerator Convection Exterior : fl_lib/Thermal/Thermal Elements/Convective Heat Transfer  area=exterior_surface_area m^2  heat_tr_coeff=natural_convection_coefficient W/(m^2 * K)  T_specify=off  T_priority=High  T=0 K  T_nominal_specify=off  T_nominal_unit=K  T_nominal_value=1  Q_specify=off  Q_priority=High  Q=0 J/s  Q_nominal_specify=off  Q_nominal_unit=W  Q_nominal_value=1
  Refrigerator Convection Interior : fl_lib/Thermal/Thermal Elements/Convective Heat Transfer  area=interior_surface_area m^2  heat_tr_coeff=natural_convection_coefficient W/(m^2 * K)  T_specify=off  T_priority=High  T=0 K  T_nominal_specify=off  T_nominal_unit=K  T_nominal_value=1  Q_specify=off  Q_priority=High  Q=0 J/s  Q_nominal_specify=off  Q_nominal_unit=W  Q_nominal_value=1
  Temperature Sensor : Subsystem
  T : PMIOPort  Side=Left
  Air : PMIOPort  Port=2  Side=Left
  S : Outport
  wires:
  Temperature Sensor/1(T) -> S/1
  connections:
  Evaporator Convection/LConn1 -- Heat Flow Sensor/RConn1
  T/RConn1 -- Heat Flow Sensor/LConn1
  Refrigerator Convection Exterior/RConn1 -- Environment Temperature/LConn1
  Refrigerator Convection Interior/LConn1 -- Evaporator Convection/RConn1 -- Temperature Sensor/LConn1 -- Air/RConn1
  Refrigerator Convection Interior/RConn1 -- Polyurethane Foam Conduction/LConn1
  Polyurethane Foam Conduction/RConn1 -- Refrigerator Convection Exterior/LConn1

== system V.1.0.SystemsmModelling/Air Conditioning System/Air Conditioner Model1/Compressor ==
  On : Inport
  Commanded Mass Flow Rate : Gain  Gain=commanded_mass_flow
  Compressor Lag : TransferFcn  Numerator=[(9/compressor_time_constant)^2]  Denominator=[1, 2*(9/compressor_time_constant), (9/compressor_time_constant)^2]
  Controlled Mass Flow Rate Source : refrigeration_lib/Controlled Mass Flow Rate Source  S=pi*pipe_diameter^2/4 m^2  L=0.1 m  mdot_specify=off  mdot_priority=High  mdot=0 kg/s  mdot_nominal_specify=off  mdot_nominal_unit=kg/s  mdot_nominal_value=1  phi_A_specify=off  phi_A_priority=High  phi_A=0 kW  phi_A_nominal_specify=off  phi_A_nominal_unit=kW  phi_A_nominal_value=1  phi_B_specify=off  phi_B_priority=High  phi_B=0 kW  phi_B_nominal_specify=off  phi_B_nominal_unit=kW  phi_B_nominal_value=1  u_AI_specify=off  u_AI_priority=High  u_AI=396.921741345 kJ/kg  u_AI_nominal_specify=off  u_AI_nominal_unit=kJ/kg  u_AI_nominal_value=1  v_A_specify=off  v_A_priority=High  v_A=0.230606289431 m^3/kg  v_A_nominal_specify=off  v_A_nominal_unit=m^3/kg  v_A_nominal_value=1  u_BI_specify=off  u_BI_priority=High  u_BI=396.921741345 kJ/kg  u_BI_nominal_specify=off  u_BI_nominal_unit=kJ/kg  u_BI_nominal_value=1  v_B_specify=off  v_B_priority=High  v_B=0.230606289431 m^3/kg  v_B_nominal_specify=off  v_B_nominal_unit=m^3/kg  v_B_nominal_value=1  u_2_specify=off  u_2_priority=High  u_2=396.921741345 kJ/kg  u_2_nominal_specify=off  u_2_nominal_unit=kJ/kg  u_2_nominal_value=1  u_3_specify=off  u_3_priority=High  u_3=396.921741345 kJ/kg  u_3_nominal_specify=off  u_3_nominal_unit=kJ/kg  u_3_nominal_value=1
      settings: InternalSimscapePortConfiguration="{\"Bottom\":[],\"Left\":[{\"id\":\"A\",\"label\":\"A\",\"type\":\"refrigeration.refrigeration\"},{\"id\":\"M\",\"label\":\"M\",\"type\":\"input\"}],\"Right\":[{\"id\":\"B\",\"label\":\"B\",\"type\":\"refrigeration.refrigeration\"},{\"id\":\"W\",\"label\":\"W\",\"type\":\"output\"}],\"Top\":[]}"
  Simulink-PS Converter : nesl_utility/Simulink-PS Converter  PhysicalDomain=network_engine_domain  SubClassName=ps_input  LeftPortType=input  RightPortType=output  PseudoPeriodic=off  Frequencies=[]  NoiseDistribution=none  NoiseParameters=[]  Unit=kg/s  AffineConversion=off  FilteringAndDerivatives=zero  SimscapeFilterOrder=1  InputFilterTimeConstant=0.001  UdotUserProvided=1
  B : PMIOPort  Side=Right
  A : PMIOPort  Port=2  Side=Left
  wires:
  Compressor Lag/1 -> Simulink-PS Converter/1
  Commanded Mass Flow Rate/1 -> Compressor Lag/1
  On/1 -> Commanded Mass Flow Rate/1
  connections:
  Controlled Mass Flow Rate Source/RConn1 -- B/RConn1
  Controlled Mass Flow Rate Source/LConn2 -- Simulink-PS Converter/RConn1
  A/RConn1 -- Controlled Mass Flow Rate Source/LConn1

== system V.1.0.SystemsmModelling/Air Conditioning System/Air Conditioner Model1/Condenser ==
  Condenser Conduction : fl_lib/Thermal/Thermal Elements/Conductive Heat Transfer  area=pi*pipe_diameter*condenser_length m^2  thickness=pipe_thickness m  th_cond=copper_conductivity W/(m*K)  T_specify=off  T_priority=High  T=0 K  T_nominal_specify=off  T_nominal_unit=K  T_nominal_value=1  Q_specify=off  Q_priority=High  Q=0 J/s  Q_nominal_specify=off  Q_nominal_unit=W  Q_nominal_value=1
  Condenser Copper : fl_lib/Thermal/Thermal Elements/Thermal Mass  mass=pi*pipe_diameter*condenser_length*pipe_thickness*copper_density kg  sp_heat=copper_specific_heat J/kg/K  T_specify=on  T_priority=High  T=environment_temperature K  T_nominal_specify=off  T_nominal_unit=K  T_nominal_value=1  Q_specify=off  Q_priority=High  Q=0 J/s  Q_nominal_specify=off  Q_nominal_unit=W  Q_nominal_value=1
  Condenser Pipe : refrigeration_lib/Pipe  L=condenser_length m  S=pi*pipe_diameter^2/4 m^2  Dh=pipe_diameter m  fs=64  La=0.1*condenser_length m  eps=15e-6 m  Re_lam=2000  Re_tur=4000  J_smooth=5 kg/m^2/s  p_0=charge_pressure MPa  T_0=-1 K  x_0=initial_quality  mdot_A_specify=off  mdot_A_priority=High  mdot_A=0 kg/s  mdot_A_nominal_specify=off  mdot_A_nominal_unit=kg/s  mdot_A_nominal_value=1  mdot_B_specify=off  mdot_B_priority=High  mdot_B=0 kg/s  mdot_B_nominal_specify=off  mdot_B_nominal_unit=kg/s  mdot_B_nominal_value=1  phi_A_specify=off  phi_A_priority=High  phi_A=0 kW  phi_A_nominal_specify=off  phi_A_nominal_unit=kW  phi_A_nominal_value=1  phi_B_specify=off  phi_B_priority=High  phi_B=0 kW  phi_B_nominal_specify=off  phi_B_nominal_unit=kW  phi_B_nominal_value=1  v_A_specify=off  v_A_priority=High  v_A=0.230606289431 m^3/kg  v_A_nominal_specify=off  v_A_nominal_unit=m^3/kg  v_A_nominal_value=1  v_B_specify=off  v_B_priority=High  v_B=0.230606289431 m^3/kg  v_B_nominal_specify=off  v_B_nominal_unit=m^3/kg  v_B_nominal_value=1  p_I_specify=off  p_I_priority=High  p_I=0.101325 MPa  p_I_nominal_specify=off  p_I_nominal_unit=MPa  p_I_nominal_value=1  u_I_specify=off  u_I_priority=High  u_I=396.921741345 kJ/kg  u_I_nominal_specify=off  u_I_nominal_unit=kJ/kg  u_I_nominal_value=1  v_I_specify=off  v_I_priority=High  v_I=0.230606289431 m^3/kg  v_I_nominal_specify=off  v_I_nominal_unit=m^3/kg  v_I_nominal_value=1  q_T_specify=off  q_T_priority=High  q_T=0 kW  q_T_nominal_specify=off  q_T_nominal_unit=kW  q_T_nominal_value=1  Ff_A_specify=off  Ff_A_priority=High  Ff_A=0 N  Ff_A_nominal_specify=off  Ff_A_nominal_unit=N  Ff_A_nominal_value=1  Ff_B_specify=off  Ff_B_priority=High  Ff_B=0 N  Ff_B_nominal_specify=off  Ff_B_nominal_unit=N  Ff_B_nominal_value=1  ev_I_specify=off  ev_I_priority=High  ev_I=1.7212095226213e+3 kJ/m^3  ev_I_nominal_specify=off  ev_I_nominal_unit=kJ/m^3  ev_I_nominal_value=1  mdot_I_specify=off  mdot_I_priority=High  mdot_I=0 kg/s  mdot_I_nominal_specify=off  mdot_I_nominal_unit=kg/s  mdot_I_nominal_value=1  Nu_I_specify=off  Nu_I_priority=High  Nu_I=0  Nu_I_nominal_specify=off  Nu_I_nominal_unit=1  Nu_I_nominal_value=1
      settings: InternalSimscapePortConfiguration="{\"Bottom\":[],\"Left\":[{\"id\":\"A\",\"label\":\"A\",\"type\":\"refrigeration.refrigeration\"},{\"id\":\"T\",\"label\":\"T\",\"type\":\"foundation.thermal.thermal\"}],\"Right\":[{\"id\":\"B\",\"label\":\"B\",\"type\":\"refrigeration.refrigeration\"}],\"Top\":[]}"
  T : PMIOPort  Side=Left
  B : PMIOPort  Port=2  Side=Left
  A : PMIOPort  Port=3  Side=Right
  connections:
  Condenser Conduction/LConn1 -- Condenser Pipe/LConn2 -- Condenser Copper/LConn1
  T/RConn1 -- Condenser Conduction/RConn1
  B/RConn1 -- Condenser Pipe/RConn1
  Condenser Pipe/LConn1 -- A/RConn1

== system V.1.0.SystemsmModelling/Air Conditioning System/Air Conditioner Model1/Control ==
  Err : Inport
  Relay : Relay  OnSwitchValue=temperature_delta  OffSwitchValue=-temperature_delta
  On : Outport
  wires:
  Err/1 -> Relay/1
  Relay/1 -> On/1

== system V.1.0.SystemsmModelling/Air Conditioning System/Air Conditioner Model1/Environment ==
  Condenser Convection : fl_lib/Thermal/Thermal Elements/Convective Heat Transfer  area=fin_area m^2  heat_tr_coeff=fin_convection_coefficient W/(m^2 * K)  T_specify=off  T_priority=High  T=0 K  T_nominal_specify=off  T_nominal_unit=K  T_nominal_value=1  Q_specify=off  Q_priority=High  Q=0 J/s  Q_nominal_specify=off  Q_nominal_unit=W  Q_nominal_value=1
  Constant : Constant  Value=environment_temperature
  Ideal Temperature Source : fl_lib/Thermal/Thermal Sources/Controlled Temperature Source
  Simulink-PS Converter : nesl_utility/Simulink-PS Converter  PhysicalDomain=network_engine_domain  SubClassName=ps_input  LeftPortType=input  RightPortType=output  PseudoPeriodic=off  Frequencies=[]  NoiseDistribution=none  NoiseParameters=[]  Unit=K  AffineConversion=off  FilteringAndDerivatives=zero  SimscapeFilterOrder=1  InputFilterTimeConstant=0.001  UdotUserProvided=1
  Thermal Reference : fl_lib/Thermal/Thermal Elements/Thermal Reference
  T : PMIOPort  Side=Left
  wires:
  Constant/1 -> Simulink-PS Converter/1
  connections:
  Condenser Convection/RConn1 -- Ideal Temperature Source/LConn1
  Condenser Convection/LConn1 -- T/RConn1
  Ideal Temperature Source/RConn1 -- Simulink-PS Converter/RConn1
  Ideal Temperature Source/RConn2 -- Thermal Reference/LConn1

== system V.1.0.SystemsmModelling/Air Conditioning System/Air Conditioner Model1/Evaporator ==
  Evaporator Conduction : fl_lib/Thermal/Thermal Elements/Conductive Heat Transfer  area=pi*pipe_diameter*evaporator_length m^2  thickness=pipe_thickness m  th_cond=copper_conductivity W/(m*K)  T_specify=off  T_priority=High  T=0 K  T_nominal_specify=off  T_nominal_unit=K  T_nominal_value=1  Q_specify=off  Q_priority=High  Q=0 J/s  Q_nominal_specify=off  Q_nominal_unit=W  Q_nominal_value=1
  Evaporator Copper : fl_lib/Thermal/Thermal Elements/Thermal Mass  mass=pi*pipe_diameter*evaporator_length*pipe_thickness*copper_density kg  sp_heat=copper_specific_heat J/kg/K  T_specify=on  T_priority=High  T=target_temperature K  T_nominal_specify=off  T_nominal_unit=K  T_nominal_value=1  Q_specify=off  Q_priority=High  Q=0 J/s  Q_nominal_specify=off  Q_nominal_unit=W  Q_nominal_value=1
  Evaporator Pipe : refrigeration_lib/Pipe  L=evaporator_length m  S=pi*pipe_diameter^2/4 m^2  Dh=pipe_diameter m  fs=64  La=0.1*evaporator_length m  eps=15e-6 m  Re_lam=2000  Re_tur=4000  J_smooth=5 kg/m^2/s  p_0=charge_pressure MPa  T_0=-1 K  x_0=initial_quality  mdot_A_specify=off  mdot_A_priority=High  mdot_A=0 kg/s  mdot_A_nominal_specify=off  mdot_A_nominal_unit=kg/s  mdot_A_nominal_value=1  mdot_B_specify=off  mdot_B_priority=High  mdot_B=0 kg/s  mdot_B_nominal_specify=off  mdot_B_nominal_unit=kg/s  mdot_B_nominal_value=1  phi_A_specify=off  phi_A_priority=High  phi_A=0 kW  phi_A_nominal_specify=off  phi_A_nominal_unit=kW  phi_A_nominal_value=1  phi_B_specify=off  phi_B_priority=High  phi_B=0 kW  phi_B_nominal_specify=off  phi_B_nominal_unit=kW  phi_B_nominal_value=1  v_A_specify=off  v_A_priority=High  v_A=0.230606289431 m^3/kg  v_A_nominal_specify=off  v_A_nominal_unit=m^3/kg  v_A_nominal_value=1  v_B_specify=off  v_B_priority=High  v_B=0.230606289431 m^3/kg  v_B_nominal_specify=off  v_B_nominal_unit=m^3/kg  v_B_nominal_value=1  p_I_specify=off  p_I_priority=High  p_I=0.101325 MPa  p_I_nominal_specify=off  p_I_nominal_unit=MPa  p_I_nominal_value=1  u_I_specify=off  u_I_priority=High  u_I=396.921741345 kJ/kg  u_I_nominal_specify=off  u_I_nominal_unit=kJ/kg  u_I_nominal_value=1  v_I_specify=off  v_I_priority=High  v_I=0.230606289431 m^3/kg  v_I_nominal_specify=off  v_I_nominal_unit=m^3/kg  v_I_nominal_value=1  q_T_specify=off  q_T_priority=High  q_T=0 kW  q_T_nominal_specify=off  q_T_nominal_unit=kW  q_T_nominal_value=1  Ff_A_specify=off  Ff_A_priority=High  Ff_A=0 N  Ff_A_nominal_specify=off  Ff_A_nominal_unit=N  Ff_A_nominal_value=1  Ff_B_specify=off  Ff_B_priority=High  Ff_B=0 N  Ff_B_nominal_specify=off  Ff_B_nominal_unit=N  Ff_B_nominal_value=1  ev_I_specify=off  ev_I_priority=High  ev_I=1.7212095226213e+3 kJ/m^3  ev_I_nominal_specify=off  ev_I_nominal_unit=kJ/m^3  ev_I_nominal_value=1  mdot_I_specify=off  mdot_I_priority=High  mdot_I=0 kg/s  mdot_I_nominal_specify=off  mdot_I_nominal_unit=kg/s  mdot_I_nominal_value=1  Nu_I_specify=off  Nu_I_priority=High  Nu_I=0  Nu_I_nominal_specify=off  Nu_I_nominal_unit=1  Nu_I_nominal_value=1
      settings: InternalSimscapePortConfiguration="{\"Bottom\":[],\"Left\":[{\"id\":\"A\",\"label\":\"A\",\"type\":\"refrigeration.refrigeration\"},{\"id\":\"T\",\"label\":\"T\",\"type\":\"foundation.thermal.thermal\"}],\"Right\":[{\"id\":\"B\",\"label\":\"B\",\"type\":\"refrigeration.refrigeration\"}],\"Top\":[]}"
  A : PMIOPort  Side=Left
  B : PMIOPort  Port=2  Side=Right
  T : PMIOPort  Port=3  Side=Right
  connections:
  Evaporator Conduction/RConn1 -- T/RConn1
  Evaporator Copper/LConn1 -- Evaporator Pipe/LConn2 -- Evaporator Conduction/LConn1
  Evaporator Pipe/RConn1 -- B/RConn1
  Evaporator Pipe/LConn1 -- A/RConn1

== system V.1.0.SystemsmModelling/Air Conditioning System/Air Conditioner Model1/Expansion Valve ==
  Controlled Local Restriction : refrigeration_lib/Controlled Local Restriction  Cd=0.7  L=0.1 m  S=pi*pipe_diameter^2/4 m^2
      settings: InternalSimscapePortConfiguration="{\"Bottom\":[],\"Left\":[{\"id\":\"A\",\"label\":\"A\",\"type\":\"refrigeration.refrigeration\"},{\"id\":\"Sr\",\"label\":\"S\",\"type\":\"input\"}],\"Right\":[{\"id\":\"B\",\"label\":\"B\",\"type\":\"refrigeration.refrigeration\"}],\"Top\":[]}"
  Cycle Sensor 4 : Subsystem
  Mass Flow Sensor : Subsystem
  Valve Control : Subsystem
  A : PMIOPort  Side=Left
  B : PMIOPort  Port=2  Side=Right
  connections:
  B/RConn1 -- Cycle Sensor 4/LConn1 -- Mass Flow Sensor/RConn1
  Controlled Local Restriction/LConn1 -- A/RConn1
  Controlled Local Restriction/RConn1 -- Mass Flow Sensor/LConn1
  Controlled Local Restriction/LConn2 -- Valve Control/LConn1
  Cycle Sensor 4/RConn1 -- Valve Control/RConn1

== system V.1.0.SystemsmModelling/Air Conditioning System/Air Conditioner Model1/Plot Properties ==

== system V.1.0.SystemsmModelling/Air Conditioning System/Air Conditioner Model1/Refrigerator Compartment ==
  Environment Temperature : Subsystem
  Evaporator Convection : fl_lib/Thermal/Thermal Elements/Convective Heat Transfer  area=interior_surface_area m^2  heat_tr_coeff=natural_convection_coefficient W/(m^2 * K)  T_specify=off  T_priority=High  T=0 K  T_nominal_specify=off  T_nominal_unit=K  T_nominal_value=1  Q_specify=off  Q_priority=High  Q=0 J/s  Q_nominal_specify=off  Q_nominal_unit=W  Q_nominal_value=1
  Heat Flow Sensor : Subsystem
  Polyurethane Foam Conduction : fl_lib/Thermal/Thermal Elements/Conductive Heat Transfer  area=interior_surface_area m^2  thickness=foam_thickness m  th_cond=foam_conductivity W/(m*K)  T_specify=off  T_priority=High  T=0 K  T_nominal_specify=off  T_nominal_unit=K  T_nominal_value=1  Q_specify=off  Q_priority=High  Q=0 J/s  Q_nominal_specify=off  Q_nominal_unit=W  Q_nominal_value=1
  Refrigerator Convection Exterior : fl_lib/Thermal/Thermal Elements/Convective Heat Transfer  area=exterior_surface_area m^2  heat_tr_coeff=natural_convection_coefficient W/(m^2 * K)  T_specify=off  T_priority=High  T=0 K  T_nominal_specify=off  T_nominal_unit=K  T_nominal_value=1  Q_specify=off  Q_priority=High  Q=0 J/s  Q_nominal_specify=off  Q_nominal_unit=W  Q_nominal_value=1
  Refrigerator Convection Interior : fl_lib/Thermal/Thermal Elements/Convective Heat Transfer  area=interior_surface_area m^2  heat_tr_coeff=natural_convection_coefficient W/(m^2 * K)  T_specify=off  T_priority=High  T=0 K  T_nominal_specify=off  T_nominal_unit=K  T_nominal_value=1  Q_specify=off  Q_priority=High  Q=0 J/s  Q_nominal_specify=off  Q_nominal_unit=W  Q_nominal_value=1
  Temperature Sensor : Subsystem
  T : PMIOPort  Side=Left
  Air : PMIOPort  Port=2  Side=Left
  S : Outport
  wires:
  Temperature Sensor/1(T) -> S/1
  connections:
  Evaporator Convection/LConn1 -- Heat Flow Sensor/RConn1
  T/RConn1 -- Heat Flow Sensor/LConn1
  Refrigerator Convection Exterior/RConn1 -- Environment Temperature/LConn1
  Refrigerator Convection Interior/LConn1 -- Evaporator Convection/RConn1 -- Temperature Sensor/LConn1 -- Air/RConn1
  Refrigerator Convection Interior/RConn1 -- Polyurethane Foam Conduction/LConn1
  Polyurethane Foam Conduction/RConn1 -- Refrigerator Convection Exterior/LConn1
